simulink model "Code4capSensor"  (R2022b)
settings: Solver=FixedStepDiscrete  StartTime=0.0  StopTime=inf  RelTol=1e-3  EnableMultiTasking=on
undefined symbols (not defined in the file): ESP, IDF, IP, TCP
libraries: esp32_io_lib x3, esp32_timer_interrupt_lib x1, esp32_device_config_lib x1
Description:
  | This model is created using Waijung 2
  | (Version: 22.12a)
  | Modified using Waijung 2
  | (Version: 22.12a)
settings Model: SimulationMode=external  Creator=mcbti  LastModifiedBy=mcbti
settings SolverCC: PositivePriorityOrder=on  AutoInsertRateTranBlk=on
settings OptimizationCC: EnhancedBackFolding=on  PassReuseOutputArgsAs=Individual arguments  ZeroExternalMemoryAtStartup=off  ZeroInternalMemoryAtStartup=off  OptimizeBlockOrder=speed  DifferentSizesBufferReuse=on  OptimizationCustomize=off  EfficientTunableParamExpr=on
settings DebuggingCC: ParameterTunabilityLossMsg=error
settings HardwareCC: ProdBitPerPointer=32  ProdBitPerSizeT=32  ProdBitPerPtrDiffT=32  ProdLargestAtomicInteger=Long  ProdLargestAtomicFloat=Double  ProdWordSize=32  ProdHWDeviceType=Cadence Design Systems (Tensilica)->Espressif Xtensa single-/dual-core 32-bit LX6 microprocessor
settings SFSimCC: MATLABDynamicMemAlloc=off
settings RTWCC: Description=Waijung 2 ESP32 target  SystemTargetFile=esp32.tlc  TemplateMakefile=esp32.tmf  RetainRTWFile=on
settings CodeAppCC: ForceParamTrailComments=on  IgnoreCustomStorageClasses=off  OperatorAnnotations=on  SimulinkDataObjDesc=on  SFDataObjDesc=on  InsertBlockDesc=on
settings STFCustomTargetCC: TargetLangStandard=C99 (ISO)  MultiwordLength=256  ModelReferenceCompliant=off  CombineOutputUpdateFcns=on  ERTCustomFileBanners=on  SupportContinuousTime=off  SupportNonInlinedSFcns=off  RemoveResetFunc=on  MATLABClassNameForMDSCustomization=Simulink.SoftwareTarget.ERTCustomization  SystemTargetFile=esp32.tlc
settings ERTTargetCC: TargetLangStandard=C99 (ISO)  ModelReferenceCompliant=off  ParMdlRefBuildCompliant=off  CompOptLevelCompliant=off  ConcurrentExecutionCompliant=off  ModelStepFunctionPrototypeControlCompliant=off  CPPClassGenCompliant=off  UseToolchainInfoCompliant=off  ExtMode=on  ExtModeStaticAlloc=on  ExtModeStaticAllocSize=2048  ExtModeMexFile=ext_wifi_comm  ExtModeMexArgs='192.168.3.20' 0 256  ERTSrcFileBannerTemplate=esp32_code_template.cgt  ERTHdrFileBannerTemplate=esp32_code_template.cgt  ERTDataSrcFileTemplate=esp32_code_template.cgt  ERTDataHdrFileTemplate=esp32_code_template.cgt  ERTCustomFileTemplate=esp32_file_process.tlc

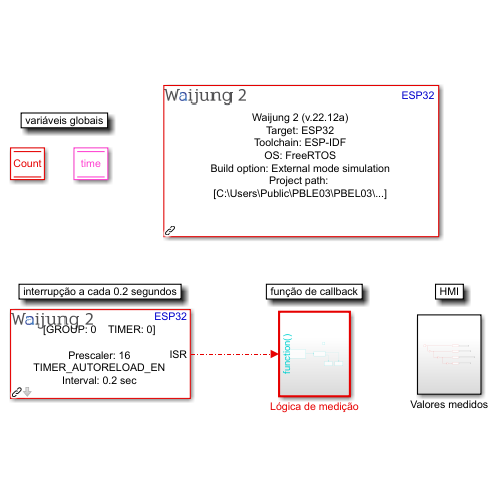
[thumbnail: Simulink's stored preview of the top-level diagram]
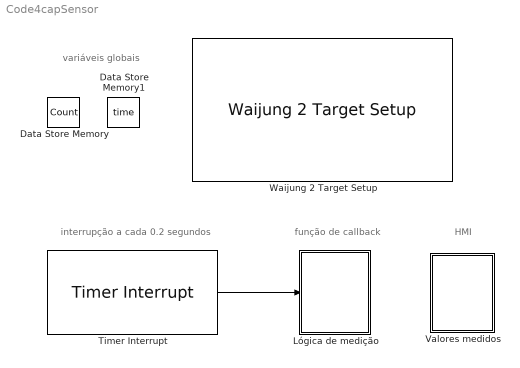
== system Code4capSensor ==
  note: HMI
  note: função de callback
  note: interrupção a cada 0.2 segundos
  note: variáveis globais
  Data Store Memory : DataStoreMemory  DataStoreName=Count  WriteAfterWriteMsg=warning  ShowAdditionalParam=off
  Data Store Memory1 : DataStoreMemory  DataStoreName=time  WriteAfterWriteMsg=warning  ShowAdditionalParam=off
  Lógica de medição : Subsystem  TreatAsAtomicUnit=on
  Timer Interrupt : esp32_timer_interrupt_lib/Timer Interrupt  timer_group=0  timer_module=0  timer_prescaler=16  timer_counter_direction=TIMER_COUNT_UP  counter_initial=0x00000000ULL  alarm=TIMER_ALARM_EN  alarm_mode=TIMER_AUTORELOAD_EN  interrupt_interval=0.2  blockid=TimerInterrupt  sampletime=-1
      settings: SourceProductName=Waijung 2 Blockset
  Valores medidos : Subsystem
  Waijung 2 Target Setup : esp32_device_config_lib/Waijung 2 Target Setup  waijungversion=22.12a  toolchain=ESP-IDF  os=FreeRTOS  sampletime=-1  simulink_managebuildsystem=on  projectpath=C:\Users\Public\PBLE03\PBEL03\ESP32\Code4capSensor_esp32_build_system  espidfpath=C:\msys32\home\skris\esp\esp-idf  buildoptions=External mode simulation  blockid=Waijung2TargetSetup  target=ESP32  defaultstacksize=2048  basepriority=0  highestpriority=10  generate_baserate_task=on  tickrate=1000  esp32target=ESP32  esp32targetdef=esp32  esp32flashsize=4MB  esp32comport=COM3  esp32baudrate=460800  esp32advancedconfig=off  esp32partitiontable=Use default waijung2 partition table  esp32partitionpath=Browse the partition table  partitionname=partitions.csv  editpartition=off  custompartitiondata={'nvs','data','nvs','','0x6000','';'phy_init','data','phy','','0x1000','';'factory','app','factory','','1M',''}  reqblocks=default  esp32custompartition={'nvs','data','nvs','','0x6000','';'phy_init','data','phy','','0x1000','';'factory','app','factory','','1M',''}  cominterface=TCP/IP  uart_module=0  baudrate=115200  tx_pin=0  rx_pin=0  com_port=9  wifimode=WIFI STA  wifissid=Rede_Loki  wifipassword=Renato.112358  deviceip=192.168.3.20  targetgateway=192.168.3.1  targetnetmask=255.255.255.0  manualdns=on  targetdnsip=8.8.8.8  targetipport=256  targetipdef=192,168,3,20  targetmaskdef=255,255,255,0  targetgatewaydef=192,168,3,1  targetdnsipdef=8,8,8,8  hosttimeout=10  hostverbose=off
      settings: SourceProductName=Waijung 2 Blockset
  wires:
  Timer Interrupt/1 -> Lógica de medição/Trigger

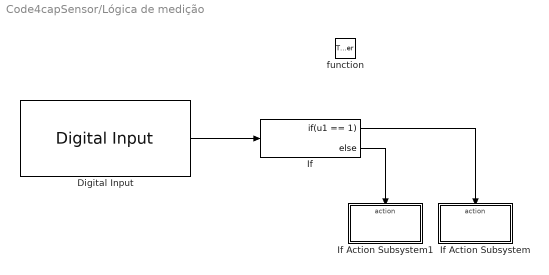
== system Code4capSensor/Lógica de medição ==
  function : TriggerPort  TriggerType=function-call  VariantControl=(inherit)
  Digital Input : esp32_io_lib/Digital Input  blockid=FunctionCallSubsystemDigitalInput  settings=Advanced  overridepin=off  pin0=off  pin1=off  pin2=off  pin3=on  pin4=off  pin5=off  pin6=off  pin7=off  pin8=off  pin9=off  pin10=off  pin11=off  pin12=off  pin13=off  pin14=off  pin15=off  pin16=off  pin17=off  pin18=off  pin19=off  pin20=off  pin21=off  pin22=off  pin23=off  pin24=off  pin25=off  pin26=off  pin27=off  pin28=off  pin29=off  pin30=off  pin31=off  pin32=off  pin33=off  pin34=off  pin35=off  pin36=off  pin37=off  pin38=off  pin39=off  pin40=off  pin41=off  pin42=off  pin43=off  pin44=off  pin45=off  pin46=off  pin47=off  pin48=off  pull_mode=None (floating)  pin_hold=Disable  deep_sleep_pin_hold=Disable  pin_array="[0  0  0  1  0  0  0  0  0  0  0  0  0  0  0  0  0  0  0  0  0  0  0  0  0  0  0  0  0  0  0  0  0  0  0  0  0  0  0  0  0  0  0  0  0  0  0  0  0]"  inport_num=1  pin_hold_define=off  pull_mode_define=GPIO_FLOATING  deep_sleep_pin_hold_define=off  pin_string=((1ULL<<3))  numpins=49  sampletime=-1
      settings: SourceProductName=Waijung 2 Blockset
  If : If  IfExpression=u1 == 1
  If Action Subsystem : Subsystem  TreatAsAtomicUnit=on
  If Action Subsystem1 : Subsystem  TreatAsAtomicUnit=on
  wires:
  If/2 -> If Action Subsystem1/Action
  Digital Input/1 -> If/1
  If/1 -> If Action Subsystem/Action

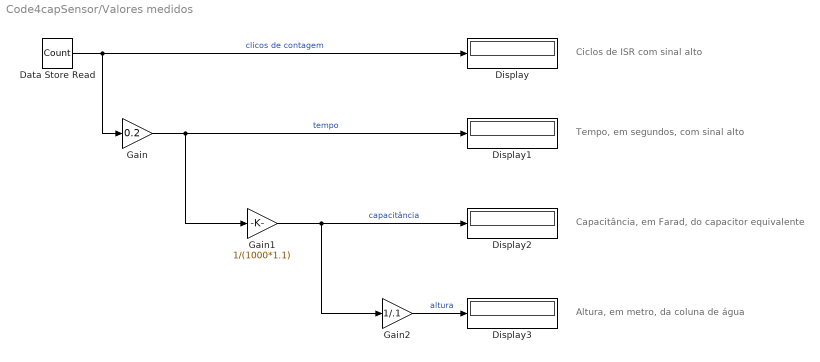
== system Code4capSensor/Valores medidos ==
  note: Ciclos de ISR com sinal alto
  note: Tempo, em segundos, com sinal alto
  note: Capacitância, em Farad, do capacitor equivalente
  note: Altura, em metro, da coluna de água
  Data Store Read : DataStoreRead  DataStoreName=Count  IndexOptions=Index vector (dialog)  Indices=1  OutputSizes=1
  Display{,1..3} (4 alike) : Display
  Gain : Gain  Gain=0.2
  Gain1 : Gain  Gain=1/(1000*1.1)
  Gain2 : Gain  Gain=1/.1
  wires:
  Gain1/1 -> Gain2/1, Display2/1  "capacitância"
  Gain2/1 -> Display3/1  "altura"
  Data Store Read/1 -> Gain/1, Display/1  "clicos de contagem"
  Gain/1 -> Gain1/1, Display1/1  "tempo"

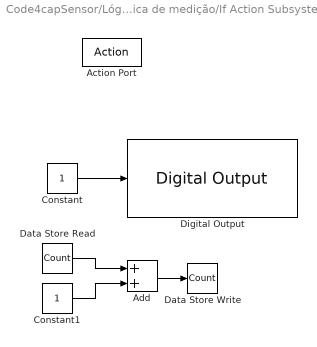
== system Code4capSensor/Lógica de medição/If Action Subsystem ==
  Action Port : ActionPort  ActionPortLabel=if(u1 == 1)
  Add : Sum
  Constant : Constant  SampleTime=-1
  Constant1 : Constant
  Data Store Read : DataStoreRead  DataStoreName=Count  IndexOptions=Index vector (dialog)  Indices=1  OutputSizes=1
  Data Store Write : DataStoreWrite  DataStoreName=Count  IndexOptions=Index vector (dialog)  Indices=1  OutputSizes=1
  Digital Output : esp32_io_lib/Digital Output  blockid=FunctionCallSubsystemIfActionSubsystemDigitalOutput  settings=Advanced  overridepin=off  pin0=off  pin1=off  pin2=off  pin3=off  pin4=off  pin5=on  pin6=off  pin7=off  pin8=off  pin9=off  pin10=off  pin11=off  pin12=off  pin13=off  pin14=off  pin15=off  pin16=off  pin17=off  pin18=off  pin19=off  pin20=off  pin21=off  pin22=off  pin23=off  pin24=off  pin25=off  pin26=off  pin27=off  pin28=off  pin29=off  pin30=off  pin31=off  pin32=off  pin33=off  pin34=off  pin35=off  pin36=off  pin37=off  pin38=off  pin39=off  pin40=off  pin41=off  pin42=off  pin43=off  pin44=off  pin45=off  pin46=off  pin47=off  pin48=off  pin_initialize=on  pin_mode=Push-pull  sampletime=-1  drive_capability=Normal (default)  pin_hold=Disable  deep_sleep_pin_hold=Disable  pin_array="[0  0  0  0  0  1  0  0  0  0  0  0  0  0  0  0  0  0  0  0  0  0  0  0  0  0  0  0  0  0  0  0  0  0  0  0  0  0  0  0  0  0  0  0  0  0  0  0  0]"  inport_num=1  drive_capability_define=GPIO_DRIVE_CAP_2  pin_hold_define=off  pin_mode_define=GPIO_MODE_INPUT_OUTPUT  deep_sleep_pin_hold_define=off  pin_string=((1ULL<<5))  numpins=49
      settings: SourceProductName=Waijung 2 Blockset
  wires:
  Constant/1 -> Digital Output/1
  Data Store Read/1 -> Add/1
  Constant1/1 -> Add/2
  Add/1 -> Data Store Write/1

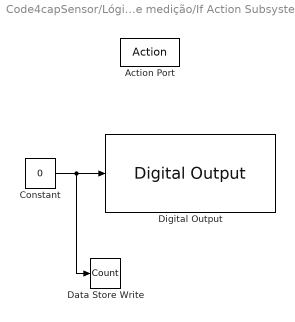
== system Code4capSensor/Lógica de medição/If Action Subsystem1 ==
  Action Port : ActionPort  ActionPortLabel=else
  Constant : Constant  Value=0  SampleTime=-1
  Data Store Write : DataStoreWrite  DataStoreName=Count  IndexOptions=Index vector (dialog)  Indices=1  OutputSizes=1
  Digital Output : esp32_io_lib/Digital Output  blockid=FunctionCallSubsystemIfActionSubsystem1DigitalOutput  settings=Advanced  overridepin=off  pin0=off  pin1=off  pin2=off  pin3=off  pin4=off  pin5=on  pin6=off  pin7=off  pin8=off  pin9=off  pin10=off  pin11=off  pin12=off  pin13=off  pin14=off  pin15=off  pin16=off  pin17=off  pin18=off  pin19=off  pin20=off  pin21=off  pin22=off  pin23=off  pin24=off  pin25=off  pin26=off  pin27=off  pin28=off  pin29=off  pin30=off  pin31=off  pin32=off  pin33=off  pin34=off  pin35=off  pin36=off  pin37=off  pin38=off  pin39=off  pin40=off  pin41=off  pin42=off  pin43=off  pin44=off  pin45=off  pin46=off  pin47=off  pin48=off  pin_initialize=on  pin_mode=Push-pull  sampletime=-1  drive_capability=Normal (default)  pin_hold=Disable  deep_sleep_pin_hold=Disable  pin_array="[0  0  0  0  0  1  0  0  0  0  0  0  0  0  0  0  0  0  0  0  0  0  0  0  0  0  0  0  0  0  0  0  0  0  0  0  0  0  0  0  0  0  0  0  0  0  0  0  0]"  inport_num=1  drive_capability_define=GPIO_DRIVE_CAP_2  pin_hold_define=off  pin_mode_define=GPIO_MODE_INPUT_OUTPUT  deep_sleep_pin_hold_define=off  pin_string=((1ULL<<5))  numpins=49
      settings: SourceProductName=Waijung 2 Blockset
  wires:
  Constant/1 -> Data Store Write/1, Digital Output/1
